simulink model "IMC_Control"  (R2020a)
settings: Solver=FixedStepAuto  StartTime=0.0  StopTime=120  FixedStep=0.001  RelTol=1e-3
settings Model: Creator=Sergio  LastModifiedBy=Sergio

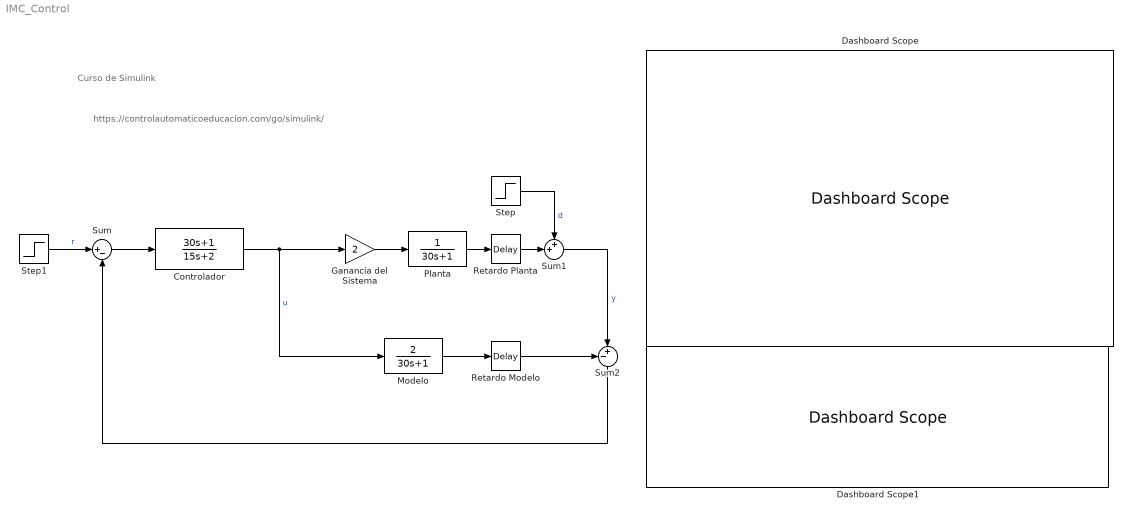
== system IMC_Control ==
  note: https://controlautomaticoeducacion.com/go/simulink/
  note: Curso de Simulink
  Controlador : TransferFcn  Numerator=[30 1]  Denominator=[15 2]
  Dashboard Scope : DashboardScope  Ymin=-0.01  Ymax=1.01
  Dashboard Scope1 : DashboardScope
  Ganancia del Sistema : Gain  Gain=2
  Modelo : TransferFcn  Numerator=[2]  Denominator=[30 1]
  Planta : TransferFcn  Denominator=[30 1]
  Retardo Modelo : TransportDelay  DelayTime=2
  Retardo Planta : TransportDelay  DelayTime=2
  Step : Step  Time=60  After=0.2  SampleTime=0
  Step1 : Step  SampleTime=0
  Sum : Sum  Inputs=|+-
  Sum1 : Sum  Inputs=++|
  Sum2 : Sum  Inputs=-+|
  wires:
  Sum/1 -> Controlador/1
  Controlador/1 -> Modelo/1, Ganancia del Sistema/1  "u"
  Planta/1 -> Retardo Planta/1
  Retardo Planta/1 -> Sum1/2
  Step/1 -> Sum1/1  "d"
  Ganancia del Sistema/1 -> Planta/1
  Step1/1 -> Sum/1  "r"
  Modelo/1 -> Retardo Modelo/1
  Retardo Modelo/1 -> Sum2/1
  Sum1/1 -> Sum2/2  "y"
  Sum2/1 -> Sum/2
